simulink model "k1visprotoIP"  (Simulink 8.5)
settings: Solver=ode45  StartTime=0.0  StopTime=10.0  RelTol=1e-3
libraries: cdsFiltCtrl x82, cdsFilt x45, cdsMuxMatrix x18, cdsEpicsOut x7, cdsEpicsBinIn x2, cdsAdcx0 x1, dac x1, simulink x1, cdsParameters x1
(part 1 of 14)
settings Model: Creator=controls  LastModifiedBy=controls
settings OptimizationCC: InitFltsAndDblsToZero=on
settings DebuggingCC: SolverPrmCheckMsg=warning  FcnCallInpInsideContextMsg=UseLocalSettings  StrictBusMsg=Warning

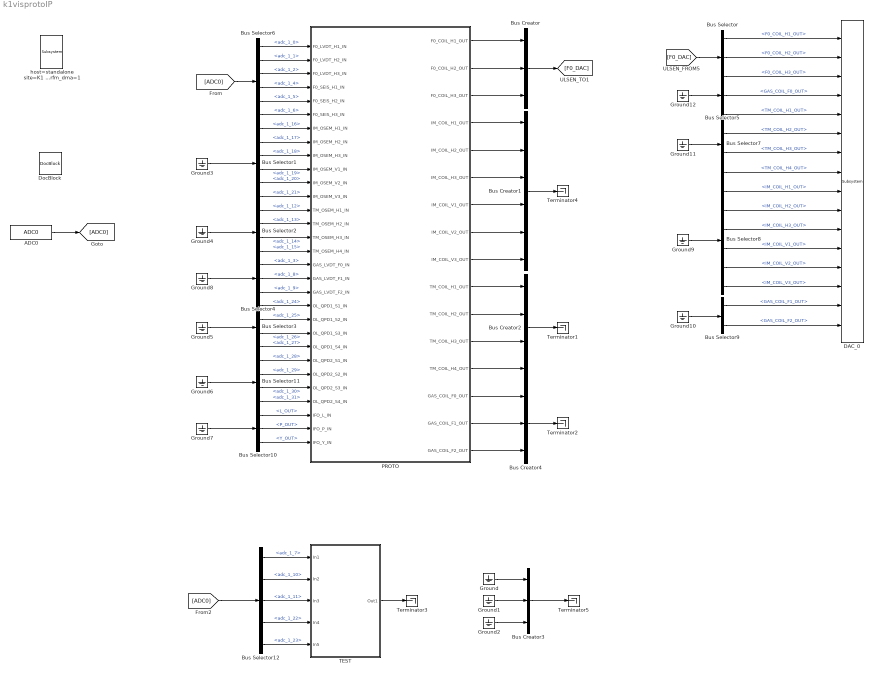
== system k1visprotoIP ==
  ADC0 : cdsAdcx0/ADC0  Tag=cdsAdc  Description=|
      | type-GSC_16AI64SSA
      | card_num=0
      settings: AttributesFormatString=%<Description>\n%<Tag>
  Bus Creator : BusCreator  Inputs='F0_COIL_H1_OUT','F0_COIL_H2_OUT','F0_COIL_H3_OUT'
  Bus Creator1 : BusCreator  Inputs='IM_COIL_H1_OUT','IM_COIL_H2_OUT','IM_COIL_H3_OUT','IM_COIL_V1_OUT','IM_COIL_V2_OUT','IM_COIL_V3_OUT'
  Bus Creator2 : BusCreator  Inputs='TM_COIL_H1_OUT','TM_COIL_H2_OUT','TM_COIL_H3_OUT','TM_COIL_H4_OUT'
  Bus Creator3 : BusCreator  Inputs='L_OUT','P_OUT','Y_OUT'
  Bus Creator4 : BusCreator  Inputs='GAS_COIL_F0_OUT','GAS_COIL_F1_OUT','GAS_COIL_F2_OUT'
  Bus Selector : BusSelector  OutputSignals=F0_COIL_H1_OUT,F0_COIL_H2_OUT,F0_COIL_H3_OUT
  Bus Selector1 : BusSelector  Description=ADC Selector  OutputSignals=adc_1_16,adc_1_17,adc_1_18,adc_1_19,adc_1_20,adc_1_21
      settings: AttributesFormatString=%<Description>
  Bus Selector10 : BusSelector  OutputSignals=L_OUT,P_OUT,Y_OUT
      settings: AttributesFormatString=%<Description>
  Bus Selector11 : BusSelector  Description=ADC Selector  OutputSignals=adc_1_28,adc_1_29,adc_1_30,adc_1_31
      settings: AttributesFormatString=%<Description>
  Bus Selector12 : BusSelector  Description=ADC Selector  OutputSignals=adc_1_7,adc_1_10,adc_1_11,adc_1_22,adc_1_23
      settings: AttributesFormatString=%<Description>
  Bus Selector2 : BusSelector  Description=ADC Selector  OutputSignals=adc_1_12,adc_1_13,adc_1_14,adc_1_15
      settings: AttributesFormatString=%<Description>
  Bus Selector3 : BusSelector  Description=ADC Selector  OutputSignals=adc_1_24,adc_1_25,adc_1_26,adc_1_27
      settings: AttributesFormatString=%<Description>
  Bus Selector4 : BusSelector  Description=ADC Selector  OutputSignals=adc_1_3,adc_1_8,adc_1_9
      settings: AttributesFormatString=%<Description>
  Bus Selector5 : BusSelector  OutputSignals=GAS_COIL_F0_OUT
  Bus Selector6 : BusSelector  Description=ADC Selector  OutputSignals=adc_1_0,adc_1_1,adc_1_2,adc_1_4,adc_1_5,adc_1_6
      settings: AttributesFormatString=%<Description>
  Bus Selector7 : BusSelector  OutputSignals=TM_COIL_H1_OUT,TM_COIL_H2_OUT,TM_COIL_H3_OUT,TM_COIL_H4_OUT
  Bus Selector8 : BusSelector  OutputSignals=IM_COIL_H1_OUT,IM_COIL_H2_OUT,IM_COIL_H3_OUT,IM_COIL_V1_OUT,IM_COIL_V2_OUT,IM_COIL_V3_OUT
  Bus Selector9 : BusSelector  OutputSignals=GAS_COIL_F1_OUT,GAS_COIL_F2_OUT
  DAC_0 : dac/Subsystem  Description=|
      | type=GSC_16AO16,
      | card_num=0
      settings: AttributesFormatString=%<Description>
  DocBlock : simulink/Model-Wide Utilities/DocBlock  DocumentType=Text
  Ground{,1..12} (13 alike) : Ground
  PROTO : Subsystem
  TEST : Subsystem
  Terminator{1..5} (5 alike) : Terminator
  host=standalone site=K1 rate=16K dcuid=99 shmem_daq=1 specific_cpu=2 adcSlave=1 no_rfm_dma=1 : cdsParameters/Subsystem  Tag=cdsParameters  Description=|
      | SCRIPT=activateDQ.py                                                                                                                                                                                                                    
      |                                                                                                                                                                                                                                         
      | Purpose:                                                                                                                                                                                                                                
      | Provide system parameters to the FE code generator to properly configure the generated EPICS names, rep rate of the FE controller, and the Data Acquisition node ID for proper storage of data from this FE controller.                 
      |                                                                                                                                                                                                                                         
      | Useage:                                                                                                                                                                                                                                 
      | The part NAME field is used to identify the FE parameters. It must be of the form:                                                                                                                                                      
      | site=                                                                                                                                                                                                                                   
      | rate=                                                                                                                                                                                                                                   
      | dcuid=                                                                                                                                                                                                                                  
      |                                                                                                                                                                                                                                         
      | Where:                                                                                                                                                                                                                                  
      | site= argument may be H1, H2, L1, M1, G1, either as a single argument or multiple, for example site=H1,H2. These are the only names allowed. These will become the first two characters of all EPICS and signal names (for example G1:).
      |                                                                                                                                                                                                                                         
      | rate= may be 2K, 16K, 32K, or 64K                                                                                                                                                                                                       
      |                                                                                                                                                                                                                                         
      | dcuid= is site specific ie it must be unique at each site.
      settings: AttributesFormatString=%<Tag>
  wires:
  Ground4/1 -> Bus Selector2/1
  Ground8/1 -> Bus Selector4/1
  Bus Creator/1 -> [F0_DAC]
  Bus Creator1/1 -> Terminator4/1
  Bus Creator2/1 -> Terminator1/1
  Bus Creator4/1 -> Terminator2/1
  [F0_DAC] -> Bus Selector/1
  Bus Selector/1 -> DAC_0/1  "<F0_COIL_H1_OUT>"
  Bus Selector/2 -> DAC_0/2  "<F0_COIL_H2_OUT>"
  Bus Selector/3 -> DAC_0/3  "<F0_COIL_H3_OUT>"
  Ground12/1 -> Bus Selector5/1
  Bus Selector5/1 -> DAC_0/4  "<GAS_COIL_F0_OUT>"
  Ground11/1 -> Bus Selector7/1
  Bus Selector7/1 -> DAC_0/5  "<TM_COIL_H1_OUT>"
  Bus Selector7/2 -> DAC_0/6  "<TM_COIL_H2_OUT>"
  Bus Selector7/3 -> DAC_0/7  "<TM_COIL_H3_OUT>"
  Bus Selector7/4 -> DAC_0/8  "<TM_COIL_H4_OUT>"
  Ground9/1 -> Bus Selector8/1
  Bus Selector8/1 -> DAC_0/9  "<IM_COIL_H1_OUT>"
  Bus Selector8/2 -> DAC_0/10  "<IM_COIL_H2_OUT>"
  Bus Selector8/3 -> DAC_0/11  "<IM_COIL_H3_OUT>"
  Bus Selector8/4 -> DAC_0/12  "<IM_COIL_V1_OUT>"
  Bus Selector8/5 -> DAC_0/13  "<IM_COIL_V2_OUT>"
  Bus Selector8/6 -> DAC_0/14  "<IM_COIL_V3_OUT>"
  Ground10/1 -> Bus Selector9/1
  Bus Selector9/1 -> DAC_0/15  "<GAS_COIL_F1_OUT>"
  Bus Selector9/2 -> DAC_0/16  "<GAS_COIL_F2_OUT>"
  Bus Selector6/1 -> PROTO/1(F0_LVDT_H1_IN)  "<adc_1_0>"
  Bus Selector6/2 -> PROTO/2(F0_LVDT_H2_IN)  "<adc_1_1>"
  Bus Selector6/3 -> PROTO/3(F0_LVDT_H3_IN)  "<adc_1_2>"
  Bus Selector6/4 -> PROTO/4(F0_SEIS_H1_IN)  "<adc_1_4>"
  Bus Selector6/5 -> PROTO/5(F0_SEIS_H2_IN)  "<adc_1_5>"
  Bus Selector6/6 -> PROTO/6(F0_SEIS_H3_IN)  "<adc_1_6>"
  Bus Selector1/1 -> PROTO/7(IM_OSEM_H1_IN)  "<adc_1_16>"
  Bus Selector1/2 -> PROTO/8(IM_OSEM_H2_IN)  "<adc_1_17>"
  Bus Selector1/3 -> PROTO/9(IM_OSEM_H3_IN)  "<adc_1_18>"
  Bus Selector1/4 -> PROTO/10(IM_OSEM_V1_IN)  "<adc_1_19>"
  Bus Selector1/5 -> PROTO/11(IM_OSEM_V2_IN)  "<adc_1_20>"
  Bus Selector1/6 -> PROTO/12(IM_OSEM_V3_IN)  "<adc_1_21>"
  Bus Selector2/1 -> PROTO/13(TM_OSEM_H1_IN)  "<adc_1_12>"
  Bus Selector2/2 -> PROTO/14(TM_OSEM_H2_IN)  "<adc_1_13>"
  Bus Selector2/3 -> PROTO/15(TM_OSEM_H3_IN)  "<adc_1_14>"
  Bus Selector2/4 -> PROTO/16(TM_OSEM_H4_IN)  "<adc_1_15>"
  Bus Selector3/1 -> PROTO/20(OL_QPD1_S1_IN)  "<adc_1_24>"
  Bus Selector3/2 -> PROTO/21(OL_QPD1_S2_IN)  "<adc_1_25>"
  Bus Selector3/3 -> PROTO/22(OL_QPD1_S3_IN)  "<adc_1_26>"
  Bus Selector3/4 -> PROTO/23(OL_QPD1_S4_IN)  "<adc_1_27>"
  Bus Selector4/1 -> PROTO/17(GAS_LVDT_F0_IN)  "<adc_1_3>"
  Bus Selector4/2 -> PROTO/18(GAS_LVDT_F1_IN)  "<adc_1_8>"
  Bus Selector4/3 -> PROTO/19(GAS_LVDT_F2_IN)  "<adc_1_9>"
  PROTO/1(F0_COIL_H1_OUT) -> Bus Creator/1
  PROTO/2(F0_COIL_H2_OUT) -> Bus Creator/2
  PROTO/3(F0_COIL_H3_OUT) -> Bus Creator/3
  PROTO/4(IM_COIL_H1_OUT) -> Bus Creator1/1
  PROTO/5(IM_COIL_H2_OUT) -> Bus Creator1/2
  PROTO/6(IM_COIL_H3_OUT) -> Bus Creator1/3
  PROTO/7(IM_COIL_V1_OUT) -> Bus Creator1/4
  PROTO/8(IM_COIL_V2_OUT) -> Bus Creator1/5
  PROTO/9(IM_COIL_V3_OUT) -> Bus Creator1/6
  PROTO/10(TM_COIL_H1_OUT) -> Bus Creator2/1
  PROTO/11(TM_COIL_H2_OUT) -> Bus Creator2/2
  PROTO/12(TM_COIL_H3_OUT) -> Bus Creator2/3
  PROTO/13(TM_COIL_H4_OUT) -> Bus Creator2/4
  PROTO/14(GAS_COIL_F0_OUT) -> Bus Creator4/1
  PROTO/15(GAS_COIL_F1_OUT) -> Bus Creator4/2
  PROTO/16(GAS_COIL_F2_OUT) -> Bus Creator4/3
  Bus Creator3/1 -> Terminator5/1
  [ADC0] -> Bus Selector12/1
  Ground7/1 -> Bus Selector10/1
  Bus Selector10/1 -> PROTO/28(IFO_L_IN)  "<L_OUT>"
  Bus Selector10/2 -> PROTO/29(IFO_P_IN)  "<P_OUT>"
  Bus Selector10/3 -> PROTO/30(IFO_Y_IN)  "<Y_OUT>"
  Ground/1 -> Bus Creator3/1
  Ground1/1 -> Bus Creator3/2
  Ground2/1 -> Bus Creator3/3
  TEST/1(Out1) -> Terminator3/1
  Bus Selector12/5 -> TEST/5(In5)  "<adc_1_23>"
  Bus Selector12/4 -> TEST/4(In4)  "<adc_1_22>"
  Bus Selector12/1 -> TEST/1(In1)  "<adc_1_7>"
  Bus Selector12/2 -> TEST/2(In2)  "<adc_1_10>"
  Bus Selector12/3 -> TEST/3(In3)  "<adc_1_11>"
  Bus Selector11/1 -> PROTO/24(OL_QPD2_S1_IN)  "<adc_1_28>"
  Bus Selector11/2 -> PROTO/25(OL_QPD2_S2_IN)  "<adc_1_29>"
  Bus Selector11/3 -> PROTO/26(OL_QPD2_S3_IN)  "<adc_1_30>"
  Bus Selector11/4 -> PROTO/27(OL_QPD2_S4_IN)  "<adc_1_31>"
  ADC0/1 -> [ADC0]
  Ground3/1 -> Bus Selector1/1
  Ground5/1 -> Bus Selector3/1
  Ground6/1 -> Bus Selector11/1
  [ADC0] -> Bus Selector6/1

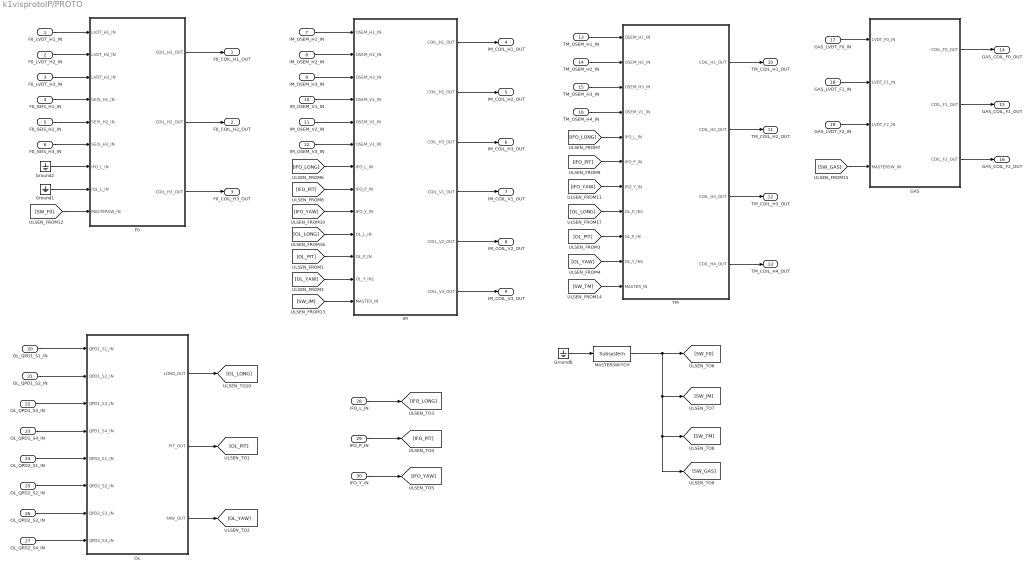
== system k1visprotoIP/PROTO ==
  F0_LVDT_H1_IN : Inport
  F0_LVDT_H2_IN : Inport  Port=2
  F0_LVDT_H3_IN : Inport  Port=3
  F0_SEIS_H1_IN : Inport  Port=4
  F0_SEIS_H2_IN : Inport  Port=5
  F0_SEIS_H3_IN : Inport  Port=6
  IM_OSEM_H1_IN : Inport  Port=7
  IM_OSEM_H2_IN : Inport  Port=8
  IM_OSEM_H3_IN : Inport  Port=9
  IM_OSEM_V1_IN : Inport  Port=10
  IM_OSEM_V2_IN : Inport  Port=11
  IM_OSEM_V3_IN : Inport  Port=12
  TM_OSEM_H1_IN : Inport  Port=13
  TM_OSEM_H2_IN : Inport  Port=14
  TM_OSEM_H3_IN : Inport  Port=15
  TM_OSEM_H4_IN : Inport  Port=16
  GAS_LVDT_F0_IN : Inport  Port=17
  GAS_LVDT_F1_IN : Inport  Port=18
  GAS_LVDT_F2_IN : Inport  Port=19
  OL_QPD1_S1_IN : Inport  Port=20
  OL_QPD1_S2_IN : Inport  Port=21
  OL_QPD1_S3_IN : Inport  Port=22
  OL_QPD1_S4_IN : Inport  Port=23
  OL_QPD2_S1_IN : Inport  Port=24
  OL_QPD2_S2_IN : Inport  Port=25
  OL_QPD2_S3_IN : Inport  Port=26
  OL_QPD2_S4_IN : Inport  Port=27
  IFO_L_IN : Inport  Port=28
  IFO_P_IN : Inport  Port=29
  IFO_Y_IN : Inport  Port=30
  F0 : Subsystem
  GAS : Subsystem
  Ground1 : Ground
  Ground2 : Ground
  Ground6 : Ground
  IM : Subsystem
  MASTERSWITCH : cdsEpicsBinIn/Subsystem  Tag=cdsEpicsBinIn  Description=|
      | Purpose:                                                                            
      | Create an EPICS binary (0 or 1) input channel to the FE realtime controls.          
      |                                                                                     
      | Operation:                                                                          
      | Outputs value from an EPICS ai record. Value is binary input (bi Epics record type).
      |                                                                                     
      | Usage:                                                                              
      | Name the part with the desired EPICS channel name.
      settings: AttributesFormatString=%<Tag>
  OL : Subsystem
  TM : Subsystem
  F0_COIL_H1_OUT : Outport
  F0_COIL_H2_OUT : Outport  Port=2
  F0_COIL_H3_OUT : Outport  Port=3
  IM_COIL_H1_OUT : Outport  Port=4
  IM_COIL_H2_OUT : Outport  Port=5
  IM_COIL_H3_OUT : Outport  Port=6
  IM_COIL_V1_OUT : Outport  Port=7
  IM_COIL_V2_OUT : Outport  Port=8
  IM_COIL_V3_OUT : Outport  Port=9
  TM_COIL_H1_OUT : Outport  Port=10
  TM_COIL_H2_OUT : Outport  Port=11
  TM_COIL_H3_OUT : Outport  Port=12
  TM_COIL_H4_OUT : Outport  Port=13
  GAS_COIL_F0_OUT : Outport  Port=14
  GAS_COIL_F1_OUT : Outport  Port=15
  GAS_COIL_F2_OUT : Outport  Port=16
  wires:
  F0/1(COIL_H1_OUT) -> F0_COIL_H1_OUT/1
  F0/2(COIL_H2_OUT) -> F0_COIL_H2_OUT/1
  F0/3(COIL_H3_OUT) -> F0_COIL_H3_OUT/1
  F0_LVDT_H1_IN/1 -> F0/1(LVDT_H1_IN)
  F0_LVDT_H2_IN/1 -> F0/2(LVDT_H2_IN)
  F0_LVDT_H3_IN/1 -> F0/3(LVDT_H3_IN)
  F0_SEIS_H1_IN/1 -> F0/4(SEIS_H1_IN)
  F0_SEIS_H2_IN/1 -> F0/5(SEIS_H2_IN)
  F0_SEIS_H3_IN/1 -> F0/6(SEIS_H3_IN)
  IM_OSEM_H1_IN/1 -> IM/1(OSEM_H1_IN)
  IM_OSEM_H2_IN/1 -> IM/2(OSEM_H2_IN)
  IM_OSEM_H3_IN/1 -> IM/3(OSEM_H3_IN)
  IM_OSEM_V1_IN/1 -> IM/4(OSEM_V1_IN)
  IM_OSEM_V2_IN/1 -> IM/5(OSEM_V2_IN)
  IM_OSEM_V3_IN/1 -> IM/6(OSEM_V3_IN)
  IM/1(COIL_H1_OUT) -> IM_COIL_H1_OUT/1
  IM/2(COIL_H2_OUT) -> IM_COIL_H2_OUT/1
  IM/3(COIL_H3_OUT) -> IM_COIL_H3_OUT/1
  IM/4(COIL_V1_OUT) -> IM_COIL_V1_OUT/1
  IM/5(COIL_V2_OUT) -> IM_COIL_V2_OUT/1
  IM/6(COIL_V3_OUT) -> IM_COIL_V3_OUT/1
  TM_OSEM_H1_IN/1 -> TM/1(OSEM_H1_IN)
  TM_OSEM_H2_IN/1 -> TM/2(OSEM_H2_IN)
  TM_OSEM_H3_IN/1 -> TM/3(OSEM_H3_IN)
  TM_OSEM_H4_IN/1 -> TM/4(OSEM_V1_IN)
  TM/1(COIL_H1_OUT) -> TM_COIL_H1_OUT/1
  TM/2(COIL_H2_OUT) -> TM_COIL_H2_OUT/1
  TM/3(COIL_H3_OUT) -> TM_COIL_H3_OUT/1
  TM/4(COIL_H4_OUT) -> TM_COIL_H4_OUT/1
  OL_QPD1_S1_IN/1 -> OL/1(QPD1_S1_IN)
  OL_QPD1_S2_IN/1 -> OL/2(QPD1_S2_IN)
  OL_QPD1_S3_IN/1 -> OL/3(QPD1_S3_IN)
  OL_QPD1_S4_IN/1 -> OL/4(QPD1_S4_IN)
  OL/2(PIT_OUT) -> [OL_PIT]
  OL/3(YAW_OUT) -> [OL_YAW]
  [OL_PIT] -> IM/11(OL_P_IN)
  [OL_YAW] -> IM/12(OL_Y_IN1)
  [OL_PIT] -> TM/9(OL_P_IN)
  [OL_YAW] -> TM/10(OL_Y_IN1)
  IFO_L_IN/1 -> [IFO_LONG]
  IFO_P_IN/1 -> [IFO_PIT]
  IFO_Y_IN/1 -> [IFO_YAW]
  Ground2/1 -> F0/7(IFO_L_IN)
  [IFO_LONG] -> IM/7(IFO_L_IN)
  [IFO_LONG] -> TM/5(IFO_L_IN)
  [IFO_PIT] -> IM/8(IFO_P_IN)
  [IFO_PIT] -> TM/6(IFO_P_IN)
  [IFO_YAW] -> IM/9(IFO_Y_IN)
  [IFO_YAW] -> TM/7(IFO_Y_IN)
  Ground6/1 -> MASTERSWITCH/1
  MASTERSWITCH/1 -> [SW_GAS], [SW_TM], [SW_IM], [SW_F0]
  [SW_F0] -> F0/9(MASTERSW_IN)
  [SW_IM] -> IM/13(MASTER_IN)
  [SW_TM] -> TM/11(MASTER_IN)
  GAS_LVDT_F0_IN/1 -> GAS/1(LVDT_F0_IN)
  [SW_GAS] -> GAS/4(MASTERSW_IN)
  GAS_LVDT_F2_IN/1 -> GAS/3(LVDT_F2_IN)
  GAS_LVDT_F1_IN/1 -> GAS/2(LVDT_F1_IN)
  GAS/1(COIL_F0_OUT) -> GAS_COIL_F0_OUT/1
  GAS/2(COIL_F1_OUT) -> GAS_COIL_F1_OUT/1
  GAS/3(COIL_F2_OUT) -> GAS_COIL_F2_OUT/1
  OL_QPD2_S1_IN/1 -> OL/5(QPD2_S1_IN)
  OL_QPD2_S2_IN/1 -> OL/6(QPD2_S2_IN)
  OL_QPD2_S3_IN/1 -> OL/7(QPD2_S3_IN)
  OL_QPD2_S4_IN/1 -> OL/8(QPD2_S4_IN)
  OL/1(LONG_OUT) -> [OL_LONG]
  [OL_LONG] -> IM/10(OL_L_IN)
  [OL_LONG] -> TM/8(OL_P_IN1)
  Ground1/1 -> F0/8(IOL_L_IN)

== system k1visprotoIP/TEST ==
  note: #DAQ Channels
      |
      | AUX1_OUT 512
  In1 : Inport
  In2 : Inport  Port=2
  In3 : Inport  Port=3
  In4 : Inport  Port=4
  In5 : Inport  Port=5
  AUX1 : cdsFilt/Subsystem  Tag=cdsFilt  Description=|
      | Purpose:                                                                                                                                                                                                                                  
      | Standard CDS IIR filter module.                                                                                                                                                                                                           
      |                                                                                                                                                                                                                                           
      | Operation:                                                                                                                                                                                                                                
      | Consists of 10 second order section IIR filters, plus a ramped gain stage. In FE code, also provides pre-defined test points and excitation channel inputs. The filter coefficients are defined in the LIGO system using the 'foton' tool.
      |                                                                                                                                                                                                                                           
      | Usage:                                                                                                                                                                                                                                    
      | Name the part with the desired filter module name.
      settings: AttributesFormatString=%<Tag>
  AUX2 : cdsFilt/Subsystem  Tag=cdsFilt  Description=|
      | Purpose:                                                                                                                                                                                                                                  
      | Standard CDS IIR filter module.                                                                                                                                                                                                           
      |                                                                                                                                                                                                                                           
      | Operation:                                                                                                                                                                                                                                
      | Consists of 10 second order section IIR filters, plus a ramped gain stage. In FE code, also provides pre-defined test points and excitation channel inputs. The filter coefficients are defined in the LIGO system using the 'foton' tool.
      |                                                                                                                                                                                                                                           
      | Usage:                                                                                                                                                                                                                                    
      | Name the part with the desired filter module name.
      settings: AttributesFormatString=%<Tag>
  AUX3 : cdsFilt/Subsystem  Tag=cdsFilt  Description=|
      | Purpose:                                                                                                                                                                                                                                  
      | Standard CDS IIR filter module.                                                                                                                                                                                                           
      |                                                                                                                                                                                                                                           
      | Operation:                                                                                                                                                                                                                                
      | Consists of 10 second order section IIR filters, plus a ramped gain stage. In FE code, also provides pre-defined test points and excitation channel inputs. The filter coefficients are defined in the LIGO system using the 'foton' tool.
      |                                                                                                                                                                                                                                           
      | Usage:                                                                                                                                                                                                                                    
      | Name the part with the desired filter module name.
      settings: AttributesFormatString=%<Tag>
  AUX4 : cdsFilt/Subsystem  Tag=cdsFilt  Description=|
      | Purpose:                                                                                                                                                                                                                                  
      | Standard CDS IIR filter module.                                                                                                                                                                                                           
      |                                                                                                                                                                                                                                           
      | Operation:                                                                                                                                                                                                                                
      | Consists of 10 second order section IIR filters, plus a ramped gain stage. In FE code, also provides pre-defined test points and excitation channel inputs. The filter coefficients are defined in the LIGO system using the 'foton' tool.
      |                                                                                                                                                                                                                                           
      | Usage:                                                                                                                                                                                                                                    
      | Name the part with the desired filter module name.
      settings: AttributesFormatString=%<Tag>
  AUX5 : cdsFilt/Subsystem  Tag=cdsFilt  Description=|
      | Purpose:                                                                                                                                                                                                                                  
      | Standard CDS IIR filter module.                                                                                                                                                                                                           
      |                                                                                                                                                                                                                                           
      | Operation:                                                                                                                                                                                                                                
      | Consists of 10 second order section IIR filters, plus a ramped gain stage. In FE code, also provides pre-defined test points and excitation channel inputs. The filter coefficients are defined in the LIGO system using the 'foton' tool.
      |                                                                                                                                                                                                                                           
      | Usage:                                                                                                                                                                                                                                    
      | Name the part with the desired filter module name.
      settings: AttributesFormatString=%<Tag>
  AUXMAT : cdsMuxMatrix/Subsystem  Tag=cdsMuxMatrix  Description=|
      | ADL=SUS_INMATRIX.adl                                                                
      | SCRIPT=generate_KisselButton.py 4 5 #CHANNEL# > #TARGET_DIR#/#FULL_PART_NAME#_KB.adl
      settings: AttributesFormatString=%<Tag>
  Demux : Demux  Outputs=1
  Ground : Ground
  Mux : Mux  Inputs=1
  Terminator{,1..4} (5 alike) : Terminator
  Out1 : Outport
  wires:
  In1/1 -> AUX1/1
  In2/1 -> AUX2/1
  In3/1 -> AUX3/1
  In4/1 -> AUX4/1
  In5/1 -> AUX5/1
  AUX1/1 -> Terminator/1
  AUX2/1 -> Terminator1/1
  AUX3/1 -> Terminator2/1
  AUX4/1 -> Terminator3/1
  AUX5/1 -> Terminator4/1
  Ground/1 -> Mux/1
  Mux/1 -> AUXMAT/1
  AUXMAT/1 -> Demux/1
  Demux/1 -> Out1/1

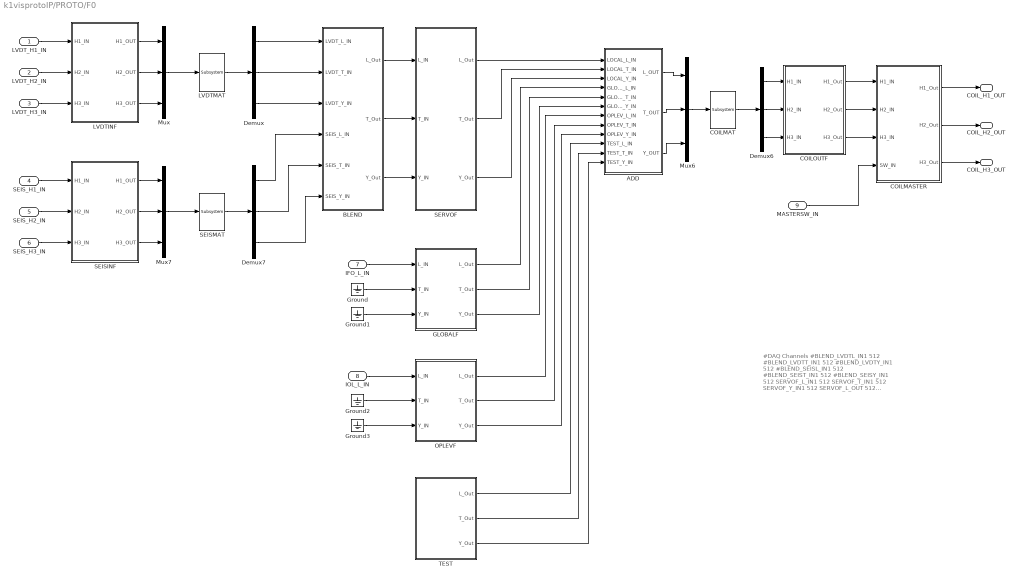
== system k1visprotoIP/PROTO/F0 ==
  note: #DAQ Channels
      |
      | #BLEND_LVDTL_IN1 512
      | #BLEND_LVDTT_IN1 512
      | #BLEND_LVDTY_IN1 512
      | #BLEND_SEISL_IN1 512
      | #BLEND_SEIST_IN1 512
      | #BLEND_SEISY_IN1 512
      | SERVOF_L_IN1 512
      | SERVOF_T_IN1 512
      | SERVOF_Y_IN1 512
      | SERVOF_L_OUT 512
      | SERVOF_T_OUT 512
      | SERVOF_Y_OUT 512
      | ADD_L_OUT 512
      | ADD_T_OUT 512
      | ADD_Y_OUT 512
      | #COILMASTER_H1_MON 512
      | #COILMASTER_H2_MON 512
      | #COILMASTER_H3_MON 512
  LVDT_H1_IN : Inport
  LVDT_H2_IN : Inport  Port=2
  LVDT_H3_IN : Inport  Port=3
  SEIS_H1_IN : Inport  Port=4
  SEIS_H2_IN : Inport  Port=5
  SEIS_H3_IN : Inport  Port=6
  IFO_L_IN : Inport  Port=7
  IOL_L_IN : Inport  Port=8
  MASTERSW_IN : Inport  Port=9
  ADD : Subsystem
  BLEND : Subsystem
  COILMASTER : Subsystem
  COILMAT : cdsMuxMatrix/Subsystem  Tag=cdsMuxMatrix  Description=|
      | ADL=SUS_INMATRIX.adl                                                                
      | SCRIPT=generate_KisselButton.py 4 5 #CHANNEL# > #TARGET_DIR#/#FULL_PART_NAME#_KB.adl
      settings: AttributesFormatString=%<Tag>
  COILOUTF : Subsystem
  Demux : Demux  Outputs=3
  Demux6 : Demux  Outputs=3
  Demux7 : Demux  Outputs=3
  GLOBALF : Subsystem
  Ground{,1..3} (4 alike) : Ground
  LVDTINF : Subsystem
  LVDTMAT : cdsMuxMatrix/Subsystem  Tag=cdsMuxMatrix  Description=|
      | ADL=SUS_INMATRIX.adl                                                                
      | SCRIPT=generate_KisselButton.py 4 5 #CHANNEL# > #TARGET_DIR#/#FULL_PART_NAME#_KB.adl
      settings: AttributesFormatString=%<Tag>
  Mux : Mux  Inputs=3
  Mux6 : Mux  Inputs=3
  Mux7 : Mux  Inputs=3
  OPLEVF : Subsystem
  SEISINF : Subsystem
  SEISMAT : cdsMuxMatrix/Subsystem  Tag=cdsMuxMatrix  Description=|
      | ADL=SUS_INMATRIX.adl                                                                
      | SCRIPT=generate_KisselButton.py 4 5 #CHANNEL# > #TARGET_DIR#/#FULL_PART_NAME#_KB.adl
      settings: AttributesFormatString=%<Tag>
  SERVOF : Subsystem
  TEST : Subsystem
  COIL_H1_OUT : Outport
  COIL_H2_OUT : Outport  Port=2
  COIL_H3_OUT : Outport  Port=3
  wires:
  LVDT_H1_IN/1 -> LVDTINF/1(H1_IN)
  LVDT_H2_IN/1 -> LVDTINF/2(H2_IN)
  LVDT_H3_IN/1 -> LVDTINF/3(H3_IN)
  LVDTINF/1(H1_OUT) -> Mux/1
  LVDTINF/2(H2_OUT) -> Mux/2
  LVDTINF/3(H3_OUT) -> Mux/3
  Mux/1 -> LVDTMAT/1
  LVDTMAT/1 -> Demux/1
  SEIS_H1_IN/1 -> SEISINF/1(H1_IN)
  Mux7/1 -> SEISMAT/1
  SEIS_H2_IN/1 -> SEISINF/2(H2_IN)
  SEIS_H3_IN/1 -> SEISINF/3(H3_IN)
  SEISINF/1(H1_OUT) -> Mux7/1
  SEISINF/3(H3_OUT) -> Mux7/3
  SEISINF/2(H2_OUT) -> Mux7/2
  SEISMAT/1 -> Demux7/1
  Demux/1 -> BLEND/1(LVDT_L_IN)
  Demux/2 -> BLEND/2(LVDT_T_IN)
  Demux/3 -> BLEND/3(LVDT_Y_IN)
  Demux7/1 -> BLEND/4(SEIS_L_IN)
  Demux7/2 -> BLEND/5(SEIS_T_IN)
  Demux7/3 -> BLEND/6(SEIS_Y_IN)
  BLEND/1(L_Out) -> SERVOF/1(L_IN)
  BLEND/2(T_Out) -> SERVOF/2(T_IN)
  BLEND/3(Y_Out) -> SERVOF/3(Y_IN)
  SERVOF/1(L_Out) -> ADD/1(LOCAL_L_IN)
  SERVOF/2(T_Out) -> ADD/2(LOCAL_T_IN)
  SERVOF/3(Y_Out) -> ADD/3(LOCAL_Y_IN)
  IFO_L_IN/1 -> GLOBALF/1(L_IN)
  GLOBALF/1(L_Out) -> ADD/4(GLOBAL_L_IN)
  GLOBALF/2(T_Out) -> ADD/5(GLOBAL_T_IN)
  GLOBALF/3(Y_Out) -> ADD/6(GLOBAL_Y_IN)
  Ground/1 -> GLOBALF/2(T_IN)
  Ground1/1 -> GLOBALF/3(Y_IN)
  ADD/1(L_OUT) -> Mux6/1
  ADD/2(T_OUT) -> Mux6/2
  ADD/3(Y_OUT) -> Mux6/3
  Mux6/1 -> COILMAT/1
  COILMAT/1 -> Demux6/1
  Demux6/1 -> COILOUTF/1(H1_IN)
  Demux6/2 -> COILOUTF/2(H2_IN)
  Demux6/3 -> COILOUTF/3(H3_IN)
  COILOUTF/1(H1_Out) -> COILMASTER/1(H1_IN)
  COILOUTF/2(H2_Out) -> COILMASTER/2(H2_IN)
  COILOUTF/3(H3_Out) -> COILMASTER/3(H3_IN)
  MASTERSW_IN/1 -> COILMASTER/4(SW_IN)
  COILMASTER/1(H1_Out) -> COIL_H1_OUT/1
  COILMASTER/2(H2_Out) -> COIL_H2_OUT/1
  COILMASTER/3(H3_Out) -> COIL_H3_OUT/1
  IOL_L_IN/1 -> OPLEVF/1(L_IN)
  Ground2/1 -> OPLEVF/2(T_IN)
  Ground3/1 -> OPLEVF/3(Y_IN)
  OPLEVF/1(L_Out) -> ADD/7(OPLEV_L_IN)
  OPLEVF/2(T_Out) -> ADD/8(OPLEV_T_IN)
  OPLEVF/3(Y_Out) -> ADD/9(OPLEV_Y_IN)
  TEST/1(L_Out) -> ADD/10(TEST_L_IN)
  TEST/2(T_Out) -> ADD/11(TEST_T_IN)
  TEST/3(Y_Out) -> ADD/12(TEST_Y_IN)

== system k1visprotoIP/PROTO/GAS ==
  LVDT_F0_IN : Inport
  LVDT_F1_IN : Inport  Port=2
  LVDT_F2_IN : Inport  Port=3
  MASTERSW_IN : Inport  Port=4
  ADD : Subsystem
  COILMASTER : Subsystem
  COILOUTF : Subsystem
  Demux1 : Demux  Outputs=3
  LVDTINF : Subsystem
  LVDTMAT : cdsMuxMatrix/Subsystem  Tag=cdsMuxMatrix  Description=|
      | ADL=SUS_INMATRIX.adl                                                                
      | SCRIPT=generate_KisselButton.py 4 5 #CHANNEL# > #TARGET_DIR#/#FULL_PART_NAME#_KB.adl
      settings: AttributesFormatString=%<Tag>
  Mux : Mux  Inputs=3
  SERVOF : Subsystem
  TEST : Subsystem
  COIL_F0_OUT : Outport
  COIL_F1_OUT : Outport  Port=2
  COIL_F2_OUT : Outport  Port=3
  wires:
  TEST/3(F2_Out) -> ADD/6(TEST_F2_IN)
  TEST/2(F1_Out) -> ADD/5(TEST_F1_IN)
  TEST/1(F0_Out) -> ADD/4(TEST_F0_IN)
  COILMASTER/3(F2_Out) -> COIL_F2_OUT/1
  COILMASTER/2(F1_Out) -> COIL_F1_OUT/1
  COILMASTER/1(F0_Out) -> COIL_F0_OUT/1
  MASTERSW_IN/1 -> COILMASTER/4(SW_IN)
  COILOUTF/3(F2_Out) -> COILMASTER/3(F2_IN)
  COILOUTF/2(F1_Out) -> COILMASTER/2(F1_IN)
  COILOUTF/1(F0_Out) -> COILMASTER/1(F0_IN)
  SERVOF/3(F2_Out) -> ADD/3(LOCAL_F2_IN)
  SERVOF/2(F1_Out) -> ADD/2(LOCAL_F1_IN)
  SERVOF/1(F0_Out) -> ADD/1(LOCAL_F0_IN)
  LVDTMAT/1 -> Demux1/1
  Mux/1 -> LVDTMAT/1
  LVDTINF/3(F2_OUT) -> Mux/3
  LVDTINF/2(F1_OUT) -> Mux/2
  LVDTINF/1(F0_OUT) -> Mux/1
  LVDT_F2_IN/1 -> LVDTINF/3(F2_IN)
  LVDT_F1_IN/1 -> LVDTINF/2(F1_IN)
  LVDT_F0_IN/1 -> LVDTINF/1(F0_IN)
  Demux1/1 -> SERVOF/1(F0_IN)
  Demux1/2 -> SERVOF/2(F1_IN)
  Demux1/3 -> SERVOF/3(F2_IN)
  ADD/1(F0_OUT) -> COILOUTF/1(F0_IN)
  ADD/2(F1_OUT) -> COILOUTF/2(F1_IN)
  ADD/3(F2_OUT) -> COILOUTF/3(F2_IN)

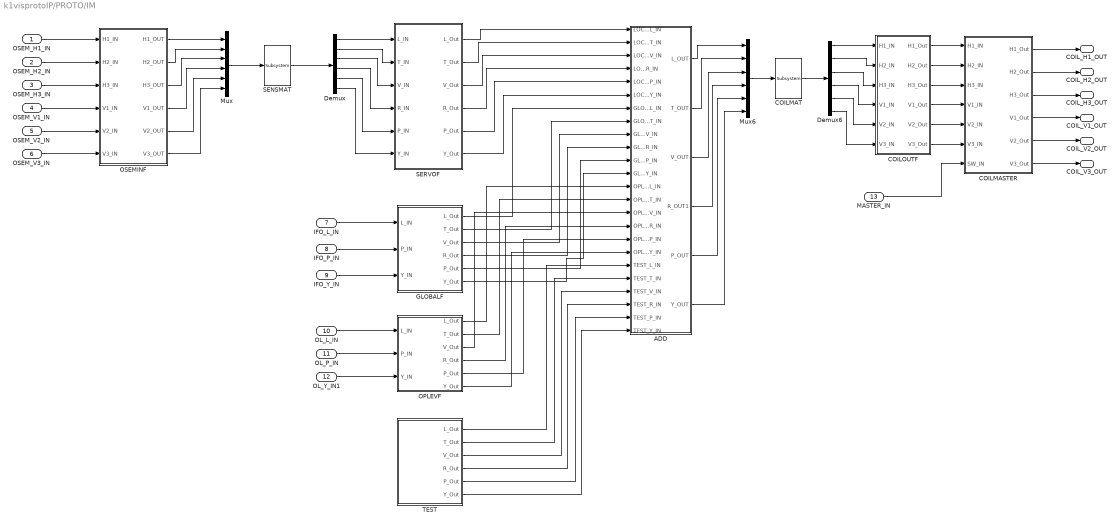
== system k1visprotoIP/PROTO/IM ==
  OSEM_H1_IN : Inport
  OSEM_H2_IN : Inport  Port=2
  OSEM_H3_IN : Inport  Port=3
  OSEM_V1_IN : Inport  Port=4
  OSEM_V2_IN : Inport  Port=5
  OSEM_V3_IN : Inport  Port=6
  IFO_L_IN : Inport  Port=7
  IFO_P_IN : Inport  Port=8
  IFO_Y_IN : Inport  Port=9
  OL_L_IN : Inport  Port=10
  OL_P_IN : Inport  Port=11
  OL_Y_IN1 : Inport  Port=12
  MASTER_IN : Inport  Port=13
  ADD : Subsystem
  COILMASTER : Subsystem
  COILMAT : cdsMuxMatrix/Subsystem  Tag=cdsMuxMatrix  Description=|
      | ADL=SUS_INMATRIX.adl                                                                
      | SCRIPT=generate_KisselButton.py 4 5 #CHANNEL# > #TARGET_DIR#/#FULL_PART_NAME#_KB.adl
      settings: AttributesFormatString=%<Tag>
  COILOUTF : Subsystem
  Demux : Demux  Outputs=6
  Demux6 : Demux  Outputs=6
  GLOBALF : Subsystem
  Mux : Mux  Inputs=6
  Mux6 : Mux  Inputs=6
  OPLEVF : Subsystem
  OSEMINF : Subsystem
  SENSMAT : cdsMuxMatrix/Subsystem  Tag=cdsMuxMatrix  Description=|
      | ADL=SUS_INMATRIX.adl                                                                
      | SCRIPT=generate_KisselButton.py 4 5 #CHANNEL# > #TARGET_DIR#/#FULL_PART_NAME#_KB.adl
      settings: AttributesFormatString=%<Tag>
  SERVOF : Subsystem
  TEST : Subsystem
  COIL_H1_OUT : Outport
  COIL_H2_OUT : Outport  Port=2
  COIL_H3_OUT : Outport  Port=3
  COIL_V1_OUT : Outport  Port=4
  COIL_V2_OUT : Outport  Port=5
  COIL_V3_OUT : Outport  Port=6
  wires:
  COILOUTF/3(H3_Out) -> COILMASTER/3(H3_IN)
  COILOUTF/2(H2_Out) -> COILMASTER/2(H2_IN)
  COILOUTF/1(H1_Out) -> COILMASTER/1(H1_IN)
  COILMAT/1 -> Demux6/1
  Mux6/1 -> COILMAT/1
  SENSMAT/1 -> Demux/1
  Mux/1 -> SENSMAT/1
  OSEMINF/3(H3_OUT) -> Mux/3
  OSEMINF/2(H2_OUT) -> Mux/2
  OSEMINF/1(H1_OUT) -> Mux/1
  OSEM_H3_IN/1 -> OSEMINF/3(H3_IN)
  OSEM_H2_IN/1 -> OSEMINF/2(H2_IN)
  OSEM_H1_IN/1 -> OSEMINF/1(H1_IN)
  OSEMINF/4(V1_OUT) -> Mux/4
  OSEMINF/5(V2_OUT) -> Mux/5
  OSEMINF/6(V3_OUT) -> Mux/6
  OSEM_V1_IN/1 -> OSEMINF/4(V1_IN)
  OSEM_V2_IN/1 -> OSEMINF/5(V2_IN)
  OSEM_V3_IN/1 -> OSEMINF/6(V3_IN)
  Demux/1 -> SERVOF/1(L_IN)
  Demux/2 -> SERVOF/2(T_IN)
  Demux/3 -> SERVOF/3(V_IN)
  Demux/4 -> SERVOF/4(R_IN)
  Demux/5 -> SERVOF/5(P_IN)
  Demux/6 -> SERVOF/6(Y_IN)
  SERVOF/1(L_Out) -> ADD/1(LOCAL_L_IN)
  SERVOF/2(T_Out) -> ADD/2(LOCAL_T_IN)
  SERVOF/3(V_Out) -> ADD/3(LOCAL_V_IN)
  SERVOF/4(R_Out) -> ADD/4(LOCAL_R_IN)
  SERVOF/5(P_Out) -> ADD/5(LOCAL_P_IN)
  SERVOF/6(Y_Out) -> ADD/6(LOCAL_Y_IN)
  IFO_L_IN/1 -> GLOBALF/1(L_IN)
  IFO_P_IN/1 -> GLOBALF/2(P_IN)
  IFO_Y_IN/1 -> GLOBALF/3(Y_IN)
  OL_P_IN/1 -> OPLEVF/2(P_IN)
  OL_Y_IN1/1 -> OPLEVF/3(Y_IN)
  TEST/1(L_Out) -> ADD/19(TEST_L_IN)
  TEST/2(T_Out) -> ADD/20(TEST_T_IN)
  TEST/3(V_Out) -> ADD/21(TEST_V_IN)
  TEST/4(R_Out) -> ADD/22(TEST_R_IN)
  TEST/5(P_Out) -> ADD/23(TEST_P_IN)
  TEST/6(Y_Out) -> ADD/24(TEST_Y_IN)
  ADD/1(L_OUT) -> Mux6/1
  ADD/2(T_OUT) -> Mux6/2
  ADD/3(V_OUT) -> Mux6/3
  ADD/4(R_OUT1) -> Mux6/4
  ADD/5(P_OUT) -> Mux6/5
  ADD/6(Y_OUT) -> Mux6/6
  Demux6/1 -> COILOUTF/1(H1_IN)
  Demux6/2 -> COILOUTF/2(H2_IN)
  Demux6/3 -> COILOUTF/3(H3_IN)
  Demux6/4 -> COILOUTF/4(V1_IN)
  Demux6/5 -> COILOUTF/5(V2_IN)
  Demux6/6 -> COILOUTF/6(V3_IN)
  COILOUTF/4(V1_Out) -> COILMASTER/4(V1_IN)
  COILOUTF/5(V2_Out) -> COILMASTER/5(V2_IN)
  COILOUTF/6(V3_Out) -> COILMASTER/6(V3_IN)
  MASTER_IN/1 -> COILMASTER/7(SW_IN)
  COILMASTER/1(H1_Out) -> COIL_H1_OUT/1
  COILMASTER/2(H2_Out) -> COIL_H2_OUT/1
  COILMASTER/3(H3_Out) -> COIL_H3_OUT/1
  COILMASTER/4(V1_Out) -> COIL_V1_OUT/1
  COILMASTER/5(V2_Out) -> COIL_V2_OUT/1
  COILMASTER/6(V3_Out) -> COIL_V3_OUT/1
  OL_L_IN/1 -> OPLEVF/1(L_IN)
  GLOBALF/4(R_Out) -> ADD/10(GLOBAL_R_IN)
  GLOBALF/1(L_Out) -> ADD/7(GLOBAL_L_IN)
  GLOBALF/2(T_Out) -> ADD/8(GLOBAL_T_IN)
  GLOBALF/3(V_Out) -> ADD/9(GLOBAL_V_IN)
  GLOBALF/5(P_Out) -> ADD/11(GLOBAL_P_IN)
  GLOBALF/6(Y_Out) -> ADD/12(GLOBAL_Y_IN)
  OPLEVF/1(L_Out) -> ADD/13(OPLEV_L_IN)
  OPLEVF/2(T_Out) -> ADD/14(OPLEV_T_IN)
  OPLEVF/3(V_Out) -> ADD/15(OPLEV_V_IN)
  OPLEVF/5(P_Out) -> ADD/17(OPLEV_P_IN)
  OPLEVF/6(Y_Out) -> ADD/18(OPLEV_Y_IN)
  OPLEVF/4(R_Out) -> ADD/16(OPLEV_R_IN)

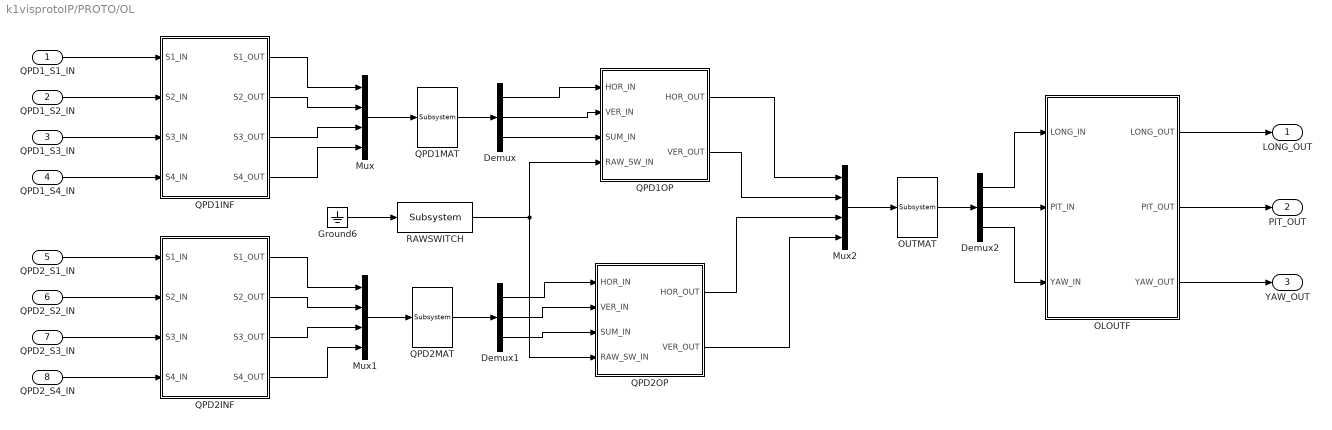
== system k1visprotoIP/PROTO/OL ==
  QPD1_S1_IN : Inport
  QPD1_S2_IN : Inport  Port=2
  QPD1_S3_IN : Inport  Port=3
  QPD1_S4_IN : Inport  Port=4
  QPD2_S1_IN : Inport  Port=5
  QPD2_S2_IN : Inport  Port=6
  QPD2_S3_IN : Inport  Port=7
  QPD2_S4_IN : Inport  Port=8
  Demux : Demux  Outputs=3
  Demux1 : Demux  Outputs=3
  Demux2 : Demux  Outputs=3
  Ground6 : Ground
  Mux : Mux
  Mux1 : Mux
  Mux2 : Mux
  OLOUTF : Subsystem
  OUTMAT : cdsMuxMatrix/Subsystem  Tag=cdsMuxMatrix  Description=|
      | ADL=SUS_INMATRIX.adl                                                                
      | SCRIPT=generate_KisselButton.py 4 5 #CHANNEL# > #TARGET_DIR#/#FULL_PART_NAME#_KB.adl
      settings: AttributesFormatString=%<Tag>
  QPD1INF : Subsystem
  QPD1MAT : cdsMuxMatrix/Subsystem  Tag=cdsMuxMatrix  Description=|
      | ADL=SUS_INMATRIX.adl                                                                
      | SCRIPT=generate_KisselButton.py 4 5 #CHANNEL# > #TARGET_DIR#/#FULL_PART_NAME#_KB.adl
      settings: AttributesFormatString=%<Tag>
  QPD1OP : Subsystem
  QPD2INF : Subsystem
  QPD2MAT : cdsMuxMatrix/Subsystem  Tag=cdsMuxMatrix  Description=|
      | ADL=SUS_INMATRIX.adl                                                                
      | SCRIPT=generate_KisselButton.py 4 5 #CHANNEL# > #TARGET_DIR#/#FULL_PART_NAME#_KB.adl
      settings: AttributesFormatString=%<Tag>
  QPD2OP : Subsystem
  RAWSWITCH : cdsEpicsBinIn/Subsystem  Tag=cdsEpicsBinIn  Description=|
      | Purpose:                                                                            
      | Create an EPICS binary (0 or 1) input channel to the FE realtime controls.          
      |                                                                                     
      | Operation:                                                                          
      | Outputs value from an EPICS ai record. Value is binary input (bi Epics record type).
      |                                                                                     
      | Usage:                                                                              
      | Name the part with the desired EPICS channel name.
      settings: AttributesFormatString=%<Tag>
  LONG_OUT : Outport
  PIT_OUT : Outport  Port=2
  YAW_OUT : Outport  Port=3
  wires:
  Mux/1 -> QPD1MAT/1
  QPD1INF/3(S3_OUT) -> Mux/3
  QPD1INF/2(S2_OUT) -> Mux/2
  QPD1INF/1(S1_OUT) -> Mux/1
  QPD1_S3_IN/1 -> QPD1INF/3(S3_IN)
  QPD1_S2_IN/1 -> QPD1INF/2(S2_IN)
  QPD1_S1_IN/1 -> QPD1INF/1(S1_IN)
  QPD1_S4_IN/1 -> QPD1INF/4(S4_IN)
  QPD1INF/4(S4_OUT) -> Mux/4
  QPD1MAT/1 -> Demux/1
  QPD2_S1_IN/1 -> QPD2INF/1(S1_IN)
  QPD2_S2_IN/1 -> QPD2INF/2(S2_IN)
  QPD2_S3_IN/1 -> QPD2INF/3(S3_IN)
  QPD2_S4_IN/1 -> QPD2INF/4(S4_IN)
  Mux1/1 -> QPD2MAT/1
  QPD2MAT/1 -> Demux1/1
  QPD2INF/1(S1_OUT) -> Mux1/1
  QPD2INF/2(S2_OUT) -> Mux1/2
  QPD2INF/3(S3_OUT) -> Mux1/3
  QPD2INF/4(S4_OUT) -> Mux1/4
  Demux/1 -> QPD1OP/1(HOR_IN)
  Demux/2 -> QPD1OP/2(VER_IN)
  Demux/3 -> QPD1OP/3(SUM_IN)
  Demux1/1 -> QPD2OP/1(HOR_IN)
  Mux2/1 -> OUTMAT/1
  OUTMAT/1 -> Demux2/1
  QPD1OP/1(HOR_OUT) -> Mux2/1
  QPD1OP/2(VER_OUT) -> Mux2/2
  QPD2OP/1(HOR_OUT) -> Mux2/3
  QPD2OP/2(VER_OUT) -> Mux2/4
  Ground6/1 -> RAWSWITCH/1
  Demux1/2 -> QPD2OP/2(VER_IN)
  Demux1/3 -> QPD2OP/3(SUM_IN)
  RAWSWITCH/1 -> QPD2OP/4(RAW_SW_IN), QPD1OP/4(RAW_SW_IN)
  OLOUTF/2(PIT_OUT) -> PIT_OUT/1
  OLOUTF/3(YAW_OUT) -> YAW_OUT/1
  OLOUTF/1(LONG_OUT) -> LONG_OUT/1
  Demux2/1 -> OLOUTF/1(LONG_IN)
  Demux2/2 -> OLOUTF/2(PIT_IN)
  Demux2/3 -> OLOUTF/3(YAW_IN)

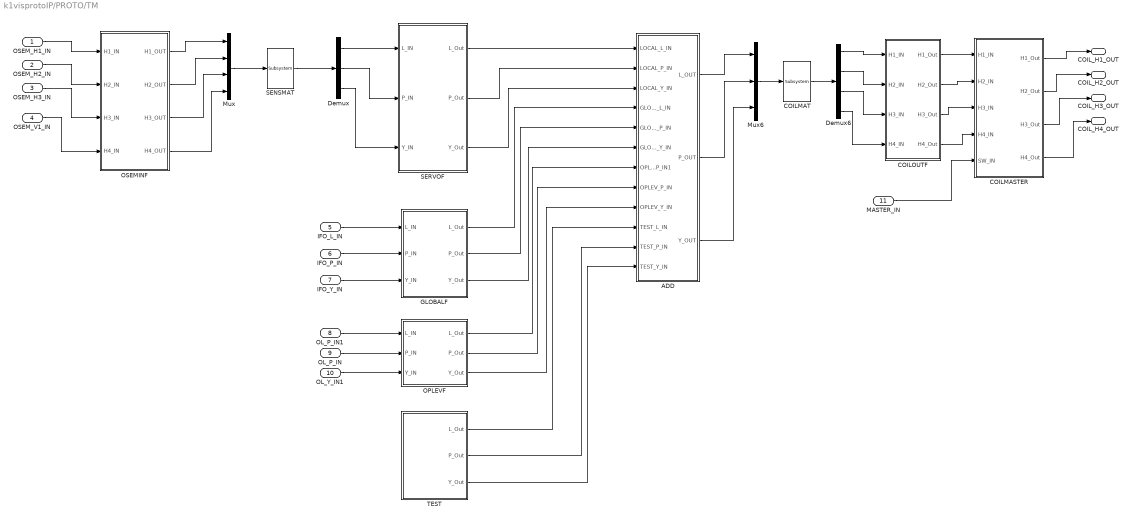
== system k1visprotoIP/PROTO/TM ==
  OSEM_H1_IN : Inport
  OSEM_H2_IN : Inport  Port=2
  OSEM_H3_IN : Inport  Port=3
  OSEM_V1_IN : Inport  Port=4
  IFO_L_IN : Inport  Port=5
  IFO_P_IN : Inport  Port=6
  IFO_Y_IN : Inport  Port=7
  OL_P_IN1 : Inport  Port=8
  OL_P_IN : Inport  Port=9
  OL_Y_IN1 : Inport  Port=10
  MASTER_IN : Inport  Port=11
  ADD : Subsystem
  COILMASTER : Subsystem
  COILMAT : cdsMuxMatrix/Subsystem  Tag=cdsMuxMatrix  Description=|
      | ADL=SUS_INMATRIX.adl                                                                
      | SCRIPT=generate_KisselButton.py 4 5 #CHANNEL# > #TARGET_DIR#/#FULL_PART_NAME#_KB.adl
      settings: AttributesFormatString=%<Tag>
  COILOUTF : Subsystem
  Demux : Demux  Outputs=3
  Demux6 : Demux
  GLOBALF : Subsystem
  Mux : Mux
  Mux6 : Mux  Inputs=3
  OPLEVF : Subsystem
  OSEMINF : Subsystem
  SENSMAT : cdsMuxMatrix/Subsystem  Tag=cdsMuxMatrix  Description=|
      | ADL=SUS_INMATRIX.adl                                                                
      | SCRIPT=generate_KisselButton.py 4 5 #CHANNEL# > #TARGET_DIR#/#FULL_PART_NAME#_KB.adl
      settings: AttributesFormatString=%<Tag>
  SERVOF : Subsystem
  TEST : Subsystem
  COIL_H1_OUT : Outport
  COIL_H2_OUT : Outport  Port=2
  COIL_H3_OUT : Outport  Port=3
  COIL_H4_OUT : Outport  Port=4
  wires:
  COILMASTER/4(H4_Out) -> COIL_H4_OUT/1
  COILMASTER/3(H3_Out) -> COIL_H3_OUT/1
  COILMASTER/2(H2_Out) -> COIL_H2_OUT/1
  COILMASTER/1(H1_Out) -> COIL_H1_OUT/1
  MASTER_IN/1 -> COILMASTER/5(SW_IN)
  COILOUTF/4(H4_Out) -> COILMASTER/4(H4_IN)
  Demux6/4 -> COILOUTF/4(H4_IN)
  Demux6/3 -> COILOUTF/3(H3_IN)
  Demux6/2 -> COILOUTF/2(H2_IN)
  Demux6/1 -> COILOUTF/1(H1_IN)
  TEST/3(Y_Out) -> ADD/12(TEST_Y_IN)
  TEST/2(P_Out) -> ADD/11(TEST_P_IN)
  TEST/1(L_Out) -> ADD/10(TEST_L_IN)
  OPLEVF/3(Y_Out) -> ADD/9(OPLEV_Y_IN)
  OPLEVF/2(P_Out) -> ADD/8(OPLEV_P_IN)
  OL_Y_IN1/1 -> OPLEVF/3(Y_IN)
  OL_P_IN/1 -> OPLEVF/2(P_IN)
  IFO_Y_IN/1 -> GLOBALF/3(Y_IN)
  IFO_P_IN/1 -> GLOBALF/2(P_IN)
  IFO_L_IN/1 -> GLOBALF/1(L_IN)
  GLOBALF/3(Y_Out) -> ADD/6(GLOBAL_Y_IN)
  GLOBALF/2(P_Out) -> ADD/5(GLOBAL_P_IN)
  GLOBALF/1(L_Out) -> ADD/4(GLOBAL_L_IN)
  SERVOF/3(Y_Out) -> ADD/3(LOCAL_Y_IN)
  SERVOF/2(P_Out) -> ADD/2(LOCAL_P_IN)
  Demux/1 -> SERVOF/1(L_IN)
  OSEM_V1_IN/1 -> OSEMINF/4(H4_IN)
  OSEMINF/4(H4_OUT) -> Mux/4
  OSEM_H1_IN/1 -> OSEMINF/1(H1_IN)
  OSEM_H2_IN/1 -> OSEMINF/2(H2_IN)
  OSEM_H3_IN/1 -> OSEMINF/3(H3_IN)
  OSEMINF/1(H1_OUT) -> Mux/1
  OSEMINF/2(H2_OUT) -> Mux/2
  OSEMINF/3(H3_OUT) -> Mux/3
  Mux/1 -> SENSMAT/1
  SENSMAT/1 -> Demux/1
  Mux6/1 -> COILMAT/1
  COILMAT/1 -> Demux6/1
  COILOUTF/1(H1_Out) -> COILMASTER/1(H1_IN)
  COILOUTF/2(H2_Out) -> COILMASTER/2(H2_IN)
  COILOUTF/3(H3_Out) -> COILMASTER/3(H3_IN)
  SERVOF/1(L_Out) -> ADD/1(LOCAL_L_IN)
  Demux/2 -> SERVOF/2(P_IN)
  Demux/3 -> SERVOF/3(Y_IN)
  ADD/1(L_OUT) -> Mux6/1
  ADD/2(P_OUT) -> Mux6/2
  ADD/3(Y_OUT) -> Mux6/3
  OPLEVF/1(L_Out) -> ADD/7(OPLEV_P_IN1)
  OL_P_IN1/1 -> OPLEVF/1(L_IN)

== system k1visprotoIP/PROTO/F0/ADD ==
  LOCAL_L_IN : Inport
  LOCAL_T_IN : Inport  Port=2
  LOCAL_Y_IN : Inport  Port=3
  GLOBAL_L_IN : Inport  Port=4
  GLOBAL_T_IN : Inport  Port=5
  GLOBAL_Y_IN : Inport  Port=6
  OPLEV_L_IN : Inport  Port=7
  OPLEV_T_IN : Inport  Port=8
  OPLEV_Y_IN : Inport  Port=9
  TEST_L_IN : Inport  Port=10
  TEST_T_IN : Inport  Port=11
  TEST_Y_IN : Inport  Port=12
  L : cdsFilt/Subsystem  Tag=cdsFilt  Description=|
      | Purpose:                                                                                                                                                                                                                                  
      | Standard CDS IIR filter module.                                                                                                                                                                                                           
      |                                                                                                                                                                                                                                           
      | Operation:                                                                                                                                                                                                                                
      | Consists of 10 second order section IIR filters, plus a ramped gain stage. In FE code, also provides pre-defined test points and excitation channel inputs. The filter coefficients are defined in the LIGO system using the 'foton' tool.
      |                                                                                                                                                                                                                                           
      | Usage:                                                                                                                                                                                                                                    
      | Name the part with the desired filter module name.
      settings: AttributesFormatString=%<Tag>
  Sum1 : Sum  Inputs=++++
  Sum2 : Sum  Inputs=++++
  Sum3 : Sum  Inputs=++++
  T : cdsFilt/Subsystem  Tag=cdsFilt  Description=|
      | Purpose:                                                                                                                                                                                                                                  
      | Standard CDS IIR filter module.                                                                                                                                                                                                           
      |                                                                                                                                                                                                                                           
      | Operation:                                                                                                                                                                                                                                
      | Consists of 10 second order section IIR filters, plus a ramped gain stage. In FE code, also provides pre-defined test points and excitation channel inputs. The filter coefficients are defined in the LIGO system using the 'foton' tool.
      |                                                                                                                                                                                                                                           
      | Usage:                                                                                                                                                                                                                                    
      | Name the part with the desired filter module name.
      settings: AttributesFormatString=%<Tag>
  Terminator1 : Terminator
  Terminator2 : Terminator
  Terminator5 : Terminator
  Y : cdsFilt/Subsystem  Tag=cdsFilt  Description=|
      | Purpose:                                                                                                                                                                                                                                  
      | Standard CDS IIR filter module.                                                                                                                                                                                                           
      |                                                                                                                                                                                                                                           
      | Operation:                                                                                                                                                                                                                                
      | Consists of 10 second order section IIR filters, plus a ramped gain stage. In FE code, also provides pre-defined test points and excitation channel inputs. The filter coefficients are defined in the LIGO system using the 'foton' tool.
      |                                                                                                                                                                                                                                           
      | Usage:                                                                                                                                                                                                                                    
      | Name the part with the desired filter module name.
      settings: AttributesFormatString=%<Tag>
  L_OUT : Outport
  T_OUT : Outport  Port=2
  Y_OUT : Outport  Port=3
  wires:
  LOCAL_L_IN/1 -> Sum1/1
  LOCAL_Y_IN/1 -> Sum3/1
  LOCAL_T_IN/1 -> Sum2/1
  GLOBAL_L_IN/1 -> Sum1/2
  GLOBAL_T_IN/1 -> Sum2/2
  GLOBAL_Y_IN/1 -> Sum3/2
  OPLEV_L_IN/1 -> Sum1/3
  OPLEV_T_IN/1 -> Sum2/3
  OPLEV_Y_IN/1 -> Sum3/3
  Sum1/1 -> L/1, L_OUT/1
  Sum2/1 -> T/1, T_OUT/1
  Sum3/1 -> Y/1, Y_OUT/1
  TEST_L_IN/1 -> Sum1/4
  TEST_T_IN/1 -> Sum2/4
  TEST_Y_IN/1 -> Sum3/4
  L/1 -> Terminator5/1
  T/1 -> Terminator1/1
  Y/1 -> Terminator2/1
